simulink model "reverb_fdn"  (R2024a)
settings: Solver=FixedStepAuto  StartTime=0.0  StopTime=5  RelTol=1e-3
values from neighbouring files (symbols this model uses):
  d1 = 5    [reverb_mooer_args.m]
  h = hadamard(4)./2    [reverb_mooer_args.m]
libraries: audiofeatures x2, dspvision x2
settings Model: Creator=fermata  LastModifiedBy=fermata
settings OptimizationCC: BlockReduction=off  ConditionallyExecuteInputs=off

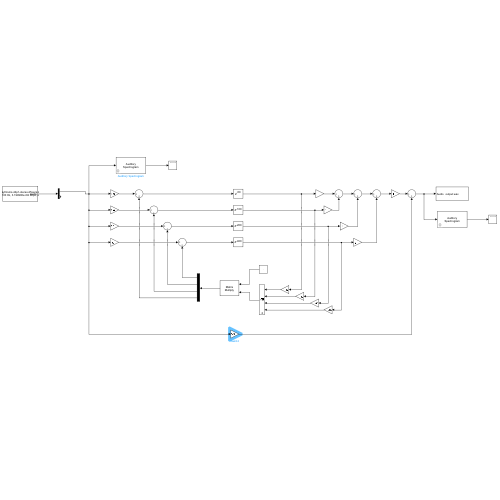
[thumbnail: Simulink's stored preview of the top-level diagram]
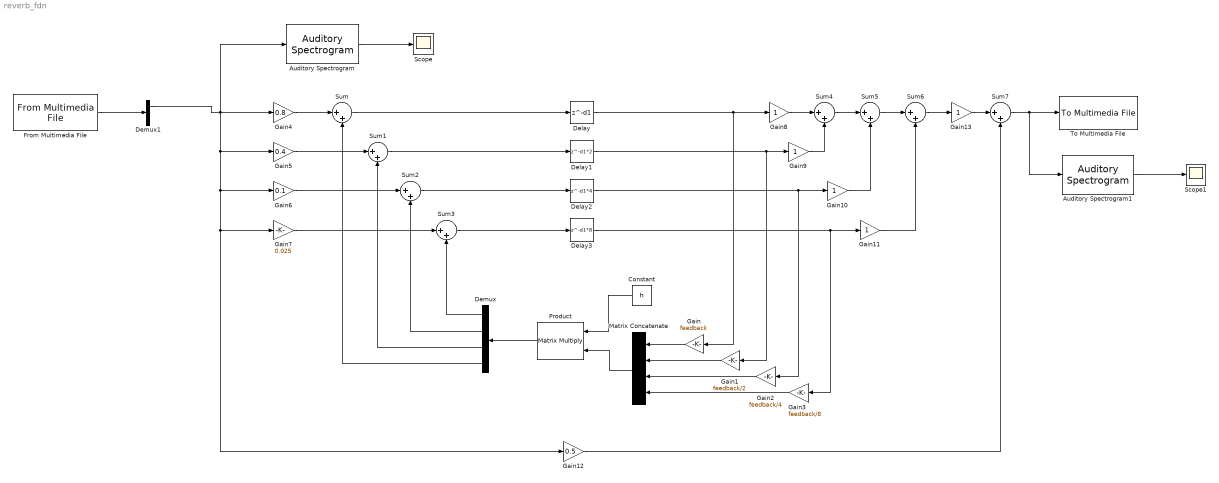
== system reverb_fdn ==
  Auditory Spectrogram : audiofeatures/Auditory Spectrogram  FrequencyScale=mel  MelStyle=oshaughnessy  AutoNumBands=on  NumBands=32  AutoFrequencyRange=on  FrequencyRange=[0, 22050]  FilterBankDesignDomain=linear  FilterBankNormalization=bandwidth  OutputFrequencyVector=off  WindowParameter=hamming(1024,'periodic')  WindowNormalization=on  OverlapLength=512  AutoFFTLength=on  FFTLength=1024  SpectrumType=magnitude  ApplyLog=off  NumHops=1  NumHopsOverlap=0  InheritSampleRate=off  SampleRate=44.1e3
  Auditory Spectrogram1 : audiofeatures/Auditory Spectrogram  FrequencyScale=mel  MelStyle=oshaughnessy  AutoNumBands=on  NumBands=32  AutoFrequencyRange=on  FrequencyRange=[0, 22050]  FilterBankDesignDomain=linear  FilterBankNormalization=bandwidth  OutputFrequencyVector=off  WindowParameter=hamming(1024,'periodic')  WindowNormalization=on  OverlapLength=512  AutoFFTLength=on  FFTLength=1024  SpectrumType=magnitude  ApplyLog=off  NumHops=1  NumHopsOverlap=0  InheritSampleRate=off  SampleRate=44.1e3
  Constant : Constant  Value=h
  Delay : Delay  DelayLength=d1  InitialCondition=0
  Delay1 : Delay  DelayLength=d1*2  InitialCondition=0
  Delay2 : Delay  DelayLength=d1*4  InitialCondition=0
  Delay3 : Delay  DelayLength=d1*8  InitialCondition=0
  Demux : Demux
  Demux1 : Demux  Outputs=2
  From Multimedia File : dspvision/From Multimedia File  inputFilename=/home/fermata/Development/Software/MATLAB/R2024a/toolbox/audio/samples/FunkyDrums-44p1-stereo-25secs.mp3  readRange=[1 Inf]  loop=on  numPlays=1  outputStreams=Audio only  videoDataType=single  audioDataType=double  inheritSampleTime=on  userDefinedSampleTime=1/1000  noAudioOutput=off  isIntensityVideo=off  fourcc=RGB  colorVideoFormat=Separate color signals  outputEOF=off  dataOrg=Column-major  audioFrameSize=1  computeAudioFrameSize=off  outSamplingMode=Sample based
      settings: LibrarySourceBlock=audiosources/From Multimedia File
  Gain : Gain  Gain=feedback
  Gain1 : Gain  Gain=feedback/2
  Gain{8..11,13} (5 alike) : Gain
  Gain12 : Gain  Gain=0.5
  Gain2 : Gain  Gain=feedback/4
  Gain3 : Gain  Gain=feedback/8
  Gain4 : Gain  Gain=0.8
  Gain5 : Gain  Gain=0.4
  Gain6 : Gain  Gain=0.1
  Gain7 : Gain  Gain=0.025
  Matrix Concatenate : Concatenate  NumInputs=4  Mode=Multidimensional array  ConcatenateDimension=2
  Product : Product  Multiplication=Matrix(*)
  Scope : Scope
  Scope1 : Scope
  Sum{,1..7} (8 alike) : Sum  Inputs=|++
  To Multimedia File : dspvision/To Multimedia File  outputFilename=/home/fermata/Development/FPGA/patatodsp/matlab/output.wav  streamSelection=Audio only  videoCompressor=None (uncompressed)  audioCompressor=None (uncompressed)  imagePorts=One multidimensional signal  fileType=WAV  audioDatatype=16-bit integer  fourcc=RGB  audioBitRate=128  audioQuality=75  videoQuality=75  mj2000CompFactor=10
      settings: LibrarySourceBlock=audiosinks/To Multimedia File
  wires:
  Auditory Spectrogram/1 -> Scope/1
  Auditory Spectrogram1/1 -> Scope1/1
  Delay/1 -> Gain8/1, Gain/1
  Delay1/1 -> Gain9/1, Gain1/1
  Delay2/1 -> Gain10/1, Gain2/1
  Delay3/1 -> Gain11/1, Gain3/1
  Matrix Concatenate/1 -> Product/2
  Constant/1 -> Product/1
  Gain/1 -> Matrix Concatenate/1
  Gain1/1 -> Matrix Concatenate/2
  Gain2/1 -> Matrix Concatenate/3
  Gain3/1 -> Matrix Concatenate/4
  Product/1 -> Demux/1
  Sum3/1 -> Delay3/1
  Sum2/1 -> Delay2/1
  Sum1/1 -> Delay1/1
  Sum/1 -> Delay/1
  Demux/2 -> Sum2/2
  Demux/3 -> Sum1/2
  Demux/4 -> Sum/2
  Sum4/1 -> Sum5/1
  Sum5/1 -> Sum6/1
  Sum7/1 -> Auditory Spectrogram1/1, To Multimedia File/1
  Gain4/1 -> Sum/1
  Gain5/1 -> Sum1/1
  Gain6/1 -> Sum2/1
  Gain7/1 -> Sum3/1
  Gain8/1 -> Sum4/1
  Gain9/1 -> Sum4/2
  Gain10/1 -> Sum5/2
  Gain11/1 -> Sum6/2
  Gain12/1 -> Sum7/2
  Sum6/1 -> Gain13/1
  Demux/1 -> Sum3/2
  From Multimedia File/1 -> Demux1/1
  Demux1/1 -> Auditory Spectrogram/1, Gain12/1, Gain7/1, Gain6/1, Gain5/1, Gain4/1
  Gain13/1 -> Sum7/1
